simulink model "parchange_task"  (Simulink 3.00)
libraries: mathlib x5, stringlib x2, speclib x1, arclib x1

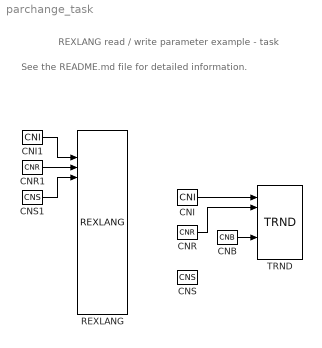
== system parchange_task ==
  note: See the README.md file for detailed information.
  note: REXLANG read / write parameter example - task
  CNB : mathlib/CNB  YCN=on
  CNI : mathlib/CNI  icn=1
  CNI1 : mathlib/CNI  icn=100
  CNR : mathlib/CNR  ycn=1
  CNR1 : mathlib/CNR  ycn=15.3
  CNS : stringlib/CNS  nmax=0
  CNS1 : stringlib/CNS  scv=rex  nmax=0
  REXLANG : speclib/REXLANG  srcname=parchange.c  srctype=1: C-like  debug=1: No check  stack=0  strs=0
  TRND : arclib/TRND  n=4  l=1000  btype=8: Double  ptype1=1: Store  ptype2=1: Store  ptype3=1: Store  ptype4=1: Store  pfac=1  afac=0  arc=0  id=1  Title=Trend Title  timesrc=1
  wires:
  CNB/1 -> TRND/5
  CNI/1 -> TRND/1
  CNI1/1 -> REXLANG/3
  CNR/1 -> TRND/2
  CNR1/1 -> REXLANG/4
  CNS1/1 -> REXLANG/5
